simulink model "powertrain_modelling_eqn0x5B10x5D"  (R2024a)
settings: Solver=VariableStepAuto  StartTime=0.0  StopTime=500  RelTol=1e-3
model workspace (MATLAB code in the model file):
  | Rw=0.32;%RADIUS OF VEHICAL(m)
  | GVM=2000;%gross vehical mass(kg)
  | GVW=GVM*9.8;%GROSS VEHICAL WEIGHT(KG)
  | CrF=0.014;%COFFICIENT OF ROLLING FRICTION
  | slope_angle=0;%slope angle in radian
  | Af=2.2;%frontal area(m^2)
  | Cd=0.25;%cofficient of drag
  | gear_ratio=9;
  | transmission_efficiency=0.95;
  | motor_eff=0.94;
  | motorcontroller_eff=0.95;
  | Bv=72;%BATTERY VOLTAGE(V)
  | Cv=3.6;%nominal voltage
  | cellcapacity=25;%cell capacity(ah)
  | lap_distance=0.787;%distance of one lap(km)
  | range=20;%range of vehical in single charge
  | time=60;%time required to complete one lap
  | air_dens=1.225;
  | We=3000; %Engine rpm
  | Engine_eff=85; %Engine efficiency
settings Model: Creator=hp  LastModifiedBy=itsme

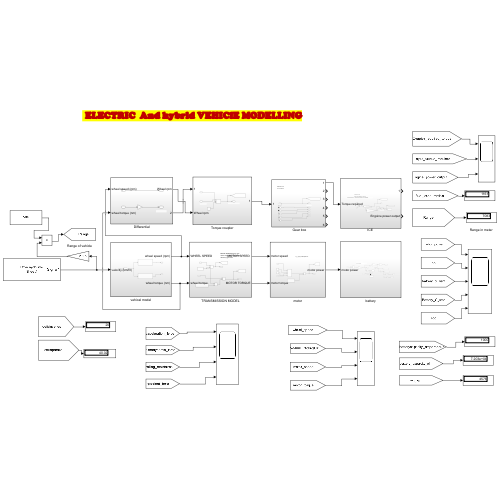
[thumbnail: Simulink's stored preview of the top-level diagram]
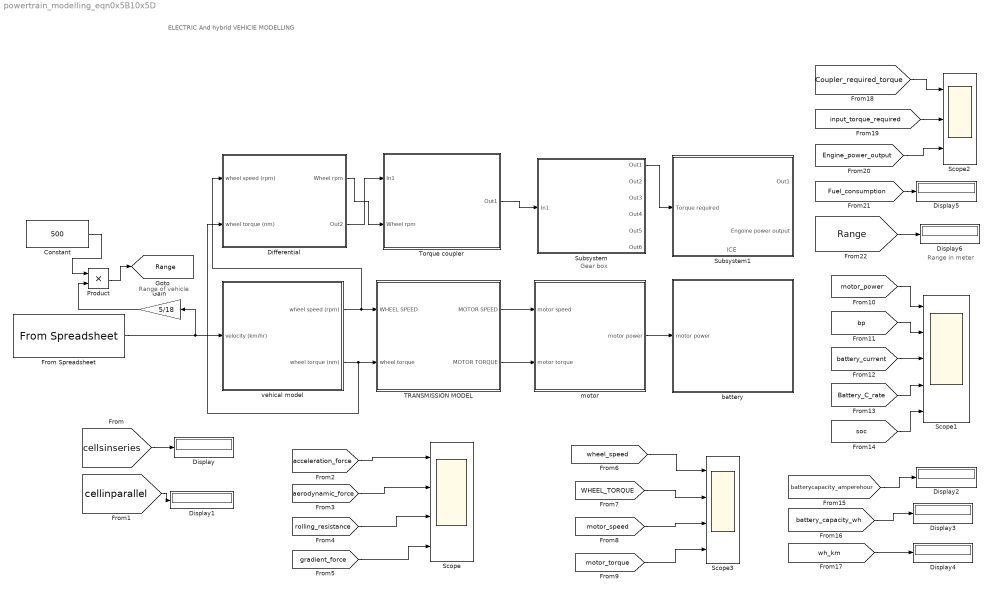
== system powertrain_modelling_eqn0x5B10x5D ==
  note: Range in meter
  note: Range of vehicle
  note: ICE
  note: Gear box
  note: ELECTRIC And hybrid VEHIClE MODELLING
  Constant : Constant  Value=500
  Differential : Subsystem
  Display{,1..6} (7 alike) : Display
  From Spreadsheet : FromSpreadsheet  FileName=Drive cycle.xlsx
  Gain : Gain  Gain=5/18
  Product : Product
  Scope : Scope  NumInputPorts=4
  Scope1 : Scope  NumInputPorts=5
  Scope2 : Scope  NumInputPorts=3
  Scope3 : Scope  NumInputPorts=4
  Subsystem : Subsystem
  Subsystem1 : Subsystem
  TRANSMISSION MODEL : Subsystem
  Torque coupler : Subsystem
  battery : Subsystem
  motor : Subsystem
  vehical model : Subsystem
  tag scope: Range=global
  wires:
  vehical model/1(wheel speed (rpm)) -> Differential/1(wheel speed (rpm)), TRANSMISSION MODEL/1(WHEEL SPEED)
  vehical model/2(wheel torque (nm)) -> Differential/2(wheel torque (nm)), TRANSMISSION MODEL/2(wheel torque)
  From Spreadsheet/1 -> Gain/1, vehical model/1(velocity (km/hr))
  TRANSMISSION MODEL/2(MOTOR TORQUE) -> motor/2(motor torque)
  TRANSMISSION MODEL/1("MOTOR SPEED ") -> motor/1(motor speed)
  motor/1(motor power) -> battery/1(motor power)
  [cellinparallel] -> Display1/1
  [cellsinseries] -> Display/1
  [acceleration_force] -> Scope/1
  [aerodynamic_force] -> Scope/2
  [rolling_resistance] -> Scope/3
  [gradient_force] -> Scope/4
  [wheel_speed] -> Scope3/1
  [WHEEL_TORQUE] -> Scope3/2
  [motor_speed] -> Scope3/3
  [motor_torque] -> Scope3/4
  [batterycapacity_amperehour] -> Display2/1
  [battery_capacity_wh] -> Display3/1
  [wh_km] -> Display4/1
  [motor_power] -> Scope1/1
  [bp] -> Scope1/2
  [battery_current] -> Scope1/3
  [Battery_C_rate] -> Scope1/4
  [soc] -> Scope1/5
  Differential/2(Out2) -> Torque coupler/1(In1)
  Torque coupler/1(Out1) -> Subsystem/1(In1)
  Subsystem/1(Out1) -> Subsystem1/1(Torque required)
  Differential/1(Wheel rpm) -> Torque coupler/2(Wheel rpm)
  [Coupler_required_torque] -> Scope2/1
  [Fuel_consumption] -> Display5/1
  [input_torque_required] -> Scope2/2
  [Engine_power_output] -> Scope2/3
  Constant/1 -> Product/1
  Product/1 -> [Range]
  [Range] -> Display6/1
  Gain/1 -> Product/2

== system powertrain_modelling_eqn0x5B10x5D/Differential ==
  note: torque required
  wheel speed (rpm) : Inport
  wheel torque (nm) : Inport  Port=2
  Gain : Gain  Gain=1/2
  Wheel rpm : Outport
  Out2 : Outport  Port=2
  wires:
  wheel speed (rpm)/1 -> Wheel rpm/1
  wheel torque (nm)/1 -> Gain/1
  Gain/1 -> Out2/1

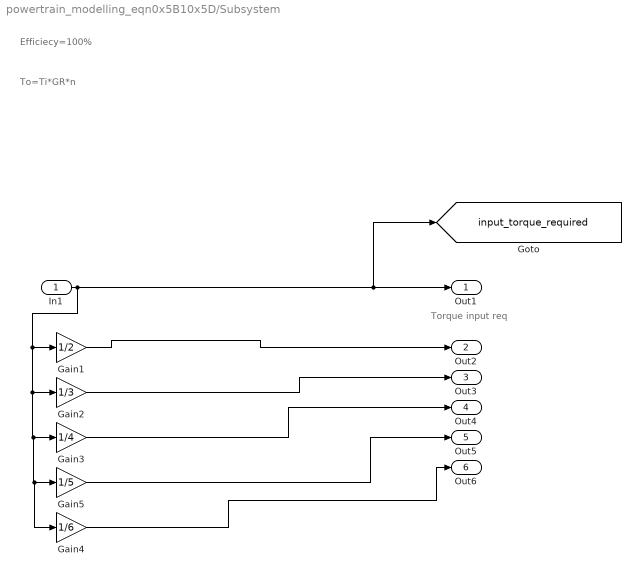
== system powertrain_modelling_eqn0x5B10x5D/Subsystem ==
  note: Torque input req
  note: To=Ti*GR*n
  note: Efficiecy=100%
  In1 : Inport
  Gain1 : Gain  Gain=1/2
  Gain2 : Gain  Gain=1/3
  Gain3 : Gain  Gain=1/4
  Gain4 : Gain  Gain=1/6
  Gain5 : Gain  Gain=1/5
  Out1 : Outport
  Out2 : Outport  Port=2
  Out3 : Outport  Port=3
  Out4 : Outport  Port=4
  Out5 : Outport  Port=5
  Out6 : Outport  Port=6
  tag scope: input_torque_required=global
  wires:
  Gain1/1 -> Out2/1
  Gain2/1 -> Out3/1
  Gain3/1 -> Out4/1
  Gain5/1 -> Out5/1
  Gain4/1 -> Out6/1
  In1/1 -> Gain4/1, Gain5/1, Gain3/1, Gain2/1, Gain1/1, [input_torque_required], Out1/1

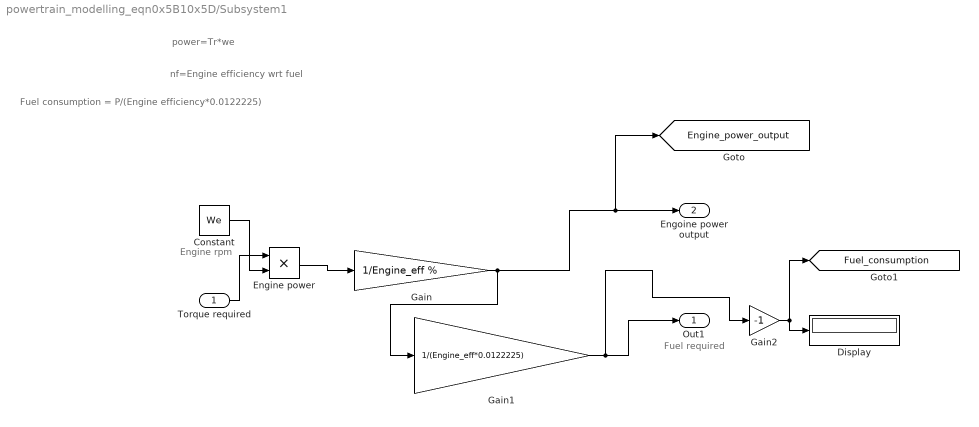
== system powertrain_modelling_eqn0x5B10x5D/Subsystem1 ==
  note: Fuel consumption = P/(Engine efficiency*0.0122225)
  note: nf=Engine efficiency wrt fuel
  note: Engine rpm
  note: power=Tr*we
  note: Fuel required
  Torque required : Inport
  Constant : Constant  Value=We
  Display : Display
  Engine power : Product
  Gain : Gain  Gain=1/Engine_eff %
  Gain1 : Gain  Gain=1/(Engine_eff*0.0122225)
  Gain2 : Gain  Gain=-1
  Out1 : Outport
  Engoine power output : Outport  Port=2
  tag scope: Engine_power_output=global, Fuel_consumption=global
  wires:
  Constant/1 -> Engine power/2
  Torque required/1 -> Engine power/1
  Engine power/1 -> Gain/1
  Gain/1 -> Gain1/1, [Engine_power_output], Engoine power output/1
  Gain1/1 -> Gain2/1, Out1/1
  Gain2/1 -> Display/1, [Fuel_consumption]

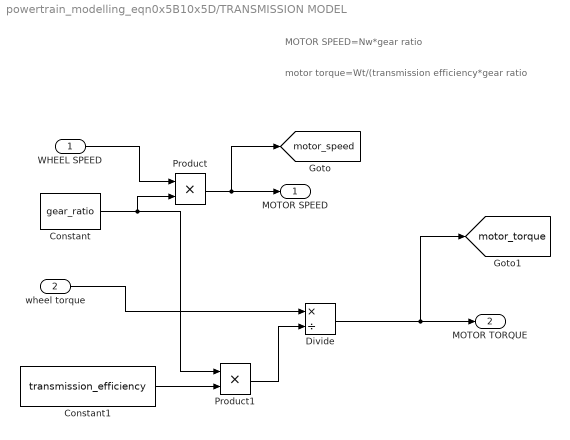
== system powertrain_modelling_eqn0x5B10x5D/TRANSMISSION MODEL ==
  note: motor torque=Wt/(transmission efficiency*gear ratio
  note: MOTOR SPEED=Nw*gear ratio
  WHEEL SPEED : Inport
  wheel torque : Inport  Port=2
  Constant : Constant  Value=gear_ratio
  Constant1 : Constant  Value=transmission_efficiency
  Divide : Product  Inputs=*/
  Product : Product
  Product1 : Product
  "MOTOR SPEED " : Outport
  MOTOR TORQUE : Outport  Port=2
  tag scope: motor_speed=global, motor_torque=global
  wires:
  WHEEL SPEED/1 -> Product/1
  Constant/1 -> Product1/1, Product/2
  Product/1 -> [motor_speed], "MOTOR SPEED "/1
  Product1/1 -> Divide/2
  Divide/1 -> [motor_torque], MOTOR TORQUE/1
  Constant1/1 -> Product1/2
  wheel torque/1 -> Divide/1

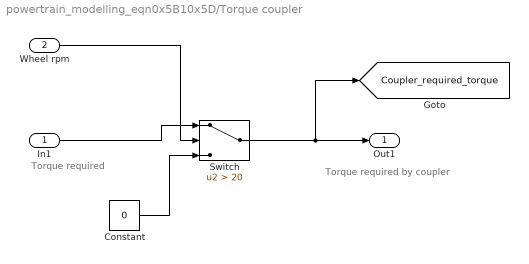
== system powertrain_modelling_eqn0x5B10x5D/Torque coupler ==
  note: Torque required by coupler
  note: Torque required
  In1 : Inport
  Wheel rpm : Inport  Port=2
  Constant : Constant  Value=0
  Switch : Switch  Criteria=u2 > Threshold  Threshold=20  SaturateOnIntegerOverflow=off  InputSameDT=off
  Out1 : Outport
  tag scope: Coupler_required_torque=global
  wires:
  In1/1 -> Switch/1
  Wheel rpm/1 -> Switch/2
  Switch/1 -> [Coupler_required_torque], Out1/1
  Constant/1 -> Switch/3

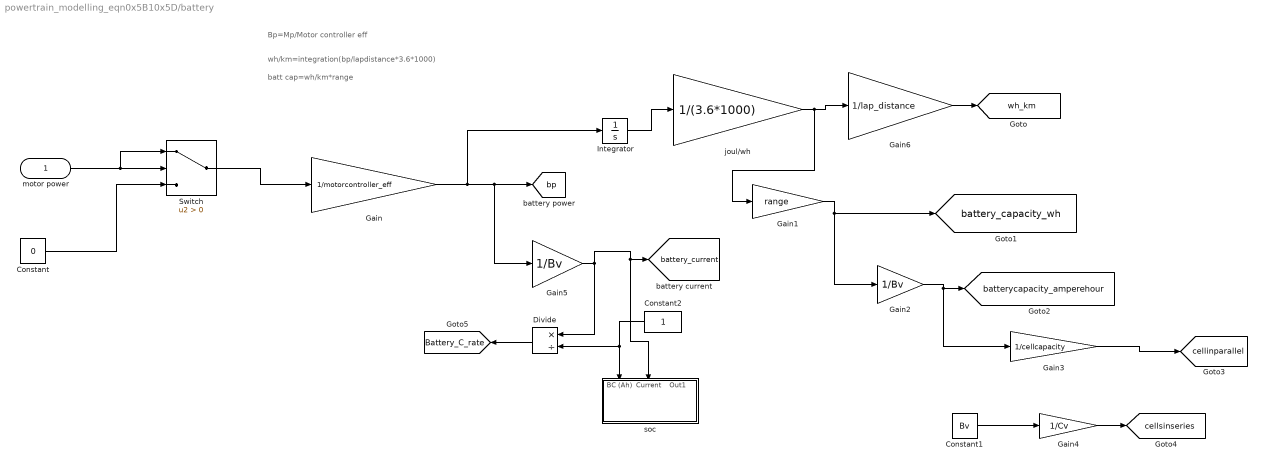
== system powertrain_modelling_eqn0x5B10x5D/battery ==
  note: batt cap=wh/km*range
  note: wh/km=integration(bp/lapdistance*3.6*1000)
  note: Bp=Mp/Motor controller eff
  motor power : Inport
  Constant : Constant  Value=0
  Constant1 : Constant  Value=Bv
  Constant2 : Constant
  Divide : Product  Inputs=*/
  Gain : Gain  Gain=1/motorcontroller_eff
  Gain1 : Gain  Gain=range
  Gain2 : Gain  Gain=1/Bv
  Gain3 : Gain  Gain=1/cellcapacity
  Gain4 : Gain  Gain=1/Cv
  Gain5 : Gain  Gain=1/Bv
  Gain6 : Gain  Gain=1/lap_distance
  Integrator : Integrator
  Switch : Switch  Criteria=u2 > Threshold  SaturateOnIntegerOverflow=off  InputSameDT=off
  joul/wh : Gain  Gain=1/(3.6*1000)
  soc : Subsystem
      settings: PortSchema="{\"entries\":[{\"content\":{\"sides\":[{\"content\":{},\"type\":\"ConnectorPlacement.EquallySpacedRectSide\",\"uuid\":\"525a52db-42a3-4186-9b86-1a9c3b979e09\"},{\"content\":{\"connectorIds\":[\"In1\",\"In2\",\"Out1\"],\"side\":\"RIGHT\"},\"type\":\"ConnectorPlacement.EquallySpacedRectSide\",\"uuid\":\"4671c8ab-09a3-4098-81cc-cb8b0c0d9d98\"},{\"content\":{\"side\":\"TOP\"},\"type\":\"ConnectorPlacement.EquallySpacedRectSide\",\"uuid\":\"72cae99d-a471-4b9e-b7ad-ba3f4cea9c19\"}]},\"type\":\"ConnectorPlacement.EquallySpacedConnector\",\"uuid\":\"a7afc5f9-2608-4223-ac98-5635804a633a\"}],\"packageUris\":[\"http://schema.mathworks.com/mf0/Connector/R2020b\"],\"version\":\"1.0\"}"
  tag scope: Battery_C_rate=global, battery_capacity_wh=global, battery_current=global, batterycapacity_amperehour=global, bp=global, cellinparallel=global, cellsinseries=global, wh_km=global
  wires:
  motor power/1 -> Switch/1, Switch/2
  Constant/1 -> Switch/3
  Switch/1 -> Gain/1
  Gain/1 -> Gain5/1, [bp], Integrator/1
  Integrator/1 -> joul/wh/1
  Gain2/1 -> Gain3/1, [batterycapacity_amperehour]
  Gain3/1 -> [cellinparallel]
  Constant1/1 -> Gain4/1
  Gain4/1 -> [cellsinseries]
  Gain5/1 -> soc/2(Current), [battery_current], Divide/1
  Divide/1 -> [Battery_C_rate]
  Constant2/1 -> soc/1(BC (Ah)), Divide/2
  Gain1/1 -> [battery_capacity_wh], Gain2/1
  joul/wh/1 -> Gain1/1, Gain6/1
  Gain6/1 -> [wh_km]

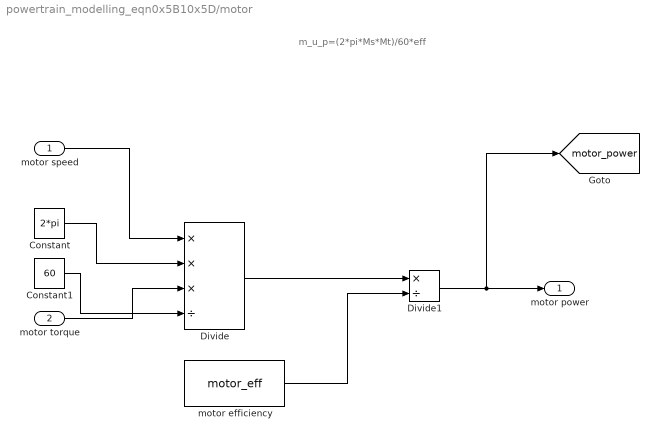
== system powertrain_modelling_eqn0x5B10x5D/motor ==
  note: m_u_p=(2*pi*Ms*Mt)/60*eff
  motor speed : Inport
  motor torque : Inport  Port=2
  Constant : Constant  Value=2*pi
  Constant1 : Constant  Value=60
  Divide : Product  Inputs=***/
  Divide1 : Product  Inputs=*/
  motor efficiency : Constant  Value=motor_eff
  motor power : Outport
  tag scope: motor_power=global
  wires:
  motor speed/1 -> Divide/1
  Constant/1 -> Divide/2
  Constant1/1 -> Divide/4
  motor torque/1 -> Divide/3
  Divide/1 -> Divide1/1
  motor efficiency/1 -> Divide1/2
  Divide1/1 -> [motor_power], motor power/1

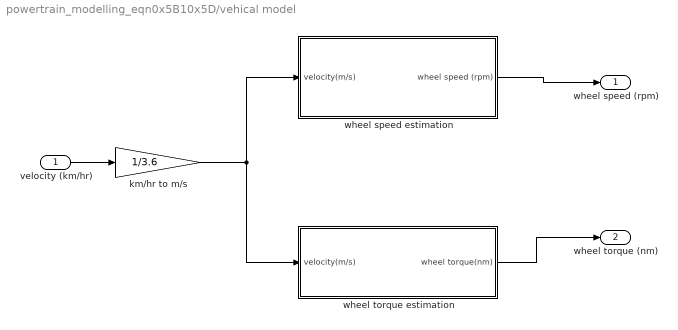
== system powertrain_modelling_eqn0x5B10x5D/vehical model ==
  velocity (km/hr) : Inport
  km/hr to m/s : Gain  Gain=1/3.6
  wheel speed estimation : Subsystem
  wheel torque estimation : Subsystem
  wheel speed (rpm) : Outport
  wheel torque (nm) : Outport  Port=2
  wires:
  velocity (km/hr)/1 -> km/hr to m/s/1
  wheel speed estimation/1(wheel speed (rpm)) -> wheel speed (rpm)/1
  wheel torque estimation/1(wheel torque(nm)) -> wheel torque (nm)/1
  km/hr to m/s/1 -> wheel speed estimation/1(velocity(m/s)), wheel torque estimation/1(velocity(m/s))

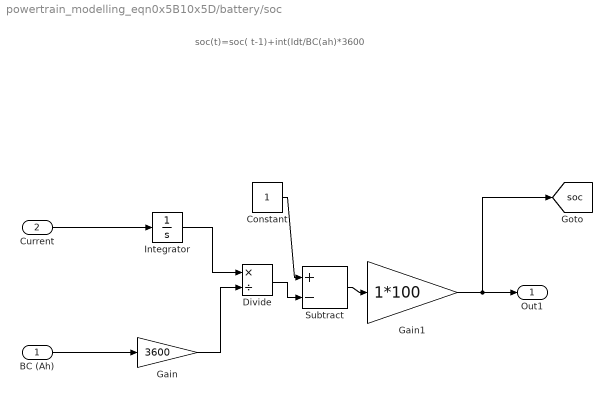
== system powertrain_modelling_eqn0x5B10x5D/battery/soc ==
  note: soc(t)=soc( t-1)+int(Idt/BC(ah)*3600
  BC (Ah) : Inport
  Current : Inport  Port=2
  Constant : Constant
  Divide : Product  Inputs=*/
  Gain : Gain  Gain=3600
  Gain1 : Gain  Gain=1*100
  Integrator : Integrator
  Subtract : Sum  Inputs=+-
  Out1 : Outport
  tag scope: soc=global
  wires:
  BC (Ah)/1 -> Gain/1
  Current/1 -> Integrator/1
  Integrator/1 -> Divide/1
  Gain/1 -> Divide/2
  Divide/1 -> Subtract/2
  Constant/1 -> Subtract/1
  Subtract/1 -> Gain1/1
  Gain1/1 -> [soc], Out1/1

== system powertrain_modelling_eqn0x5B10x5D/vehical model/wheel speed estimation ==
  note: Nw=(V*60)/(2*PI*Rw)
  velocity(m/s) : Inport
  Constant : Constant  Value=2*pi*Rw
  Divide : Product  Inputs=*/
  Gain : Gain  Gain=60
  wheel speed (rpm) : Outport
  tag scope: wheel_speed=global
  wires:
  Constant/1 -> Divide/2
  Divide/1 -> [wheel_speed], wheel speed (rpm)/1
  velocity(m/s)/1 -> Gain/1
  Gain/1 -> Divide/1

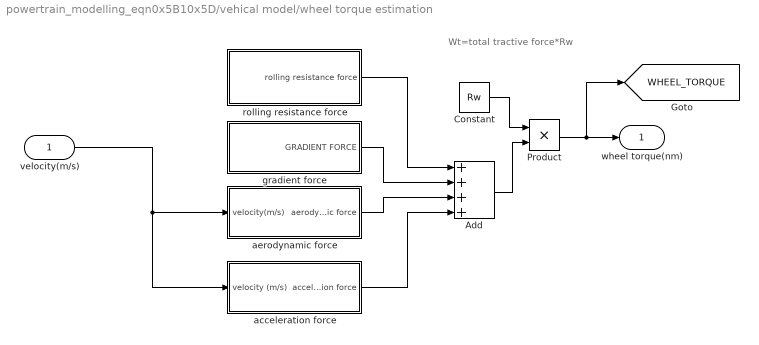
== system powertrain_modelling_eqn0x5B10x5D/vehical model/wheel torque estimation ==
  note: Wt=total tractive force*Rw
  velocity(m/s) : Inport
  Add : Sum  Inputs=++++
  Constant : Constant  Value=Rw
  Product : Product
  acceleration force : Subsystem
  aerodynamic force : Subsystem
  gradient force : Subsystem
  rolling resistance force : Subsystem
  wheel torque(nm) : Outport
  tag scope: WHEEL_TORQUE=global
  wires:
  velocity(m/s)/1 -> acceleration force/1(velocity (m/s)), aerodynamic force/1(velocity(m/s))
  rolling resistance force/1(rolling resistance force) -> Add/1
  gradient force/1(GRADIENT FORCE) -> Add/2
  aerodynamic force/1(aerodynamic force) -> Add/3
  acceleration force/1(acceleration force) -> Add/4
  Constant/1 -> Product/1
  Add/1 -> Product/2
  Product/1 -> [WHEEL_TORQUE], wheel torque(nm)/1

== system powertrain_modelling_eqn0x5B10x5D/vehical model/wheel torque estimation/acceleration force ==
  note: f acc=gvm*derivate(velocity )
  velocity (m/s) : Inport
  Constant : Constant  Value=GVM
  Derivative : Derivative
  Product : Product
  acceleration force : Outport
  tag scope: acceleration_force=global
  wires:
  velocity (m/s)/1 -> Derivative/1
  Derivative/1 -> Product/1
  Constant/1 -> Product/2
  Product/1 -> [acceleration_force], acceleration force/1

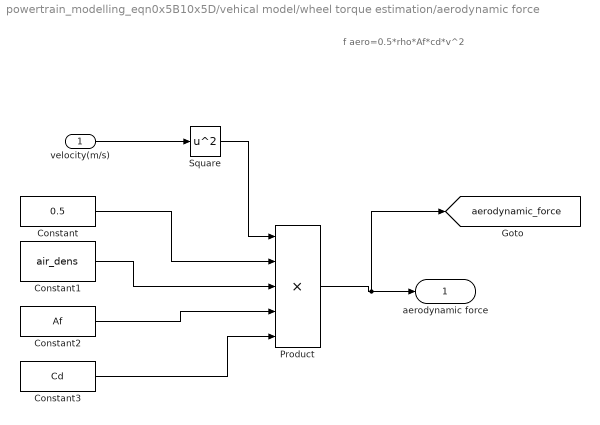
== system powertrain_modelling_eqn0x5B10x5D/vehical model/wheel torque estimation/aerodynamic force ==
  note: f aero=0.5*rho*Af*cd*v^2
  velocity(m/s) : Inport
  Constant : Constant  Value=0.5
  Constant1 : Constant  Value=air_dens
  Constant2 : Constant  Value=Af
  Constant3 : Constant  Value=Cd
  Product : Product  Inputs=5
  Square : Math  Operator=square
  aerodynamic force : Outport
  tag scope: aerodynamic_force=global
  wires:
  velocity(m/s)/1 -> Square/1
  Square/1 -> Product/1
  Constant/1 -> Product/2
  Constant1/1 -> Product/3
  Constant2/1 -> Product/4
  Constant3/1 -> Product/5
  Product/1 -> [aerodynamic_force], aerodynamic force/1

== system powertrain_modelling_eqn0x5B10x5D/vehical model/wheel torque estimation/gradient force ==
  note: F grad=GVM*SIN(THETA)
  Constant : Constant  Value=GVM
  Constant1 : Constant  Value=slope_angle
  Product : Product
  Sin : Trigonometry
  GRADIENT FORCE : Outport
  tag scope: gradient_force=global
  wires:
  Constant1/1 -> Sin/1
  Sin/1 -> Product/2
  Constant/1 -> Product/1
  Product/1 -> [gradient_force], GRADIENT FORCE/1

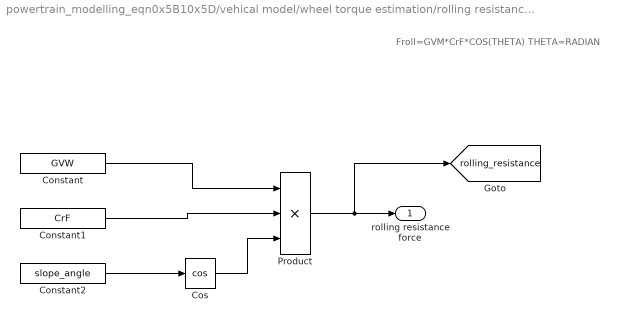
== system powertrain_modelling_eqn0x5B10x5D/vehical model/wheel torque estimation/rolling resistance force ==
  note: Froll=GVM*CrF*COS(THETA)
      | THETA=RADIAN
  Constant : Constant  Value=GVW
  Constant1 : Constant  Value=CrF
  Constant2 : Constant  Value=slope_angle
  Cos : Trigonometry  Operator=cos
  Product : Product  Inputs=3
  rolling resistance force : Outport
  tag scope: rolling_resistance=global
  wires:
  Constant2/1 -> Cos/1
  Cos/1 -> Product/3
  Constant1/1 -> Product/2
  Constant/1 -> Product/1
  Product/1 -> [rolling_resistance], rolling resistance force/1
